simulink model "roll1818002"  (R2022b)
settings: Solver=ode1  StartTime=0.0  StopTime=500  FixedStep=0.01  RelTol=1e-3
values from neighbouring files (symbols this model uses):
  Kp = 16.374    [roll201818002.m]
  Td = 0.01    [roll201818002.m]
  Ti = 150    [roll201818002.m]
settings Model: Creator=Wasif  LastModifiedBy=Wasif
settings SolverCC: ZeroCrossAlgorithm=Adaptive
settings DataIOCC: ReturnWorkspaceOutputs=off
settings DebuggingCC: IgnoredZcDiagnostic=none

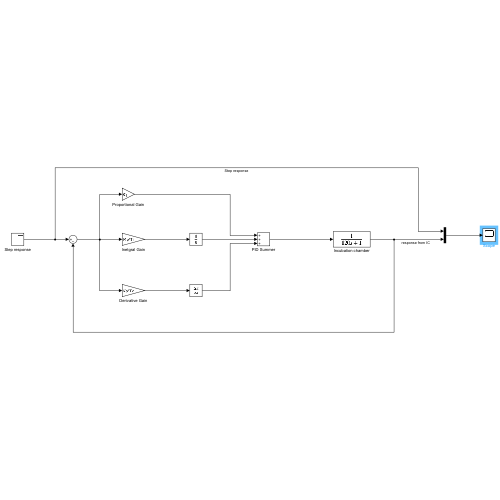
[thumbnail: Simulink's stored preview of the top-level diagram]
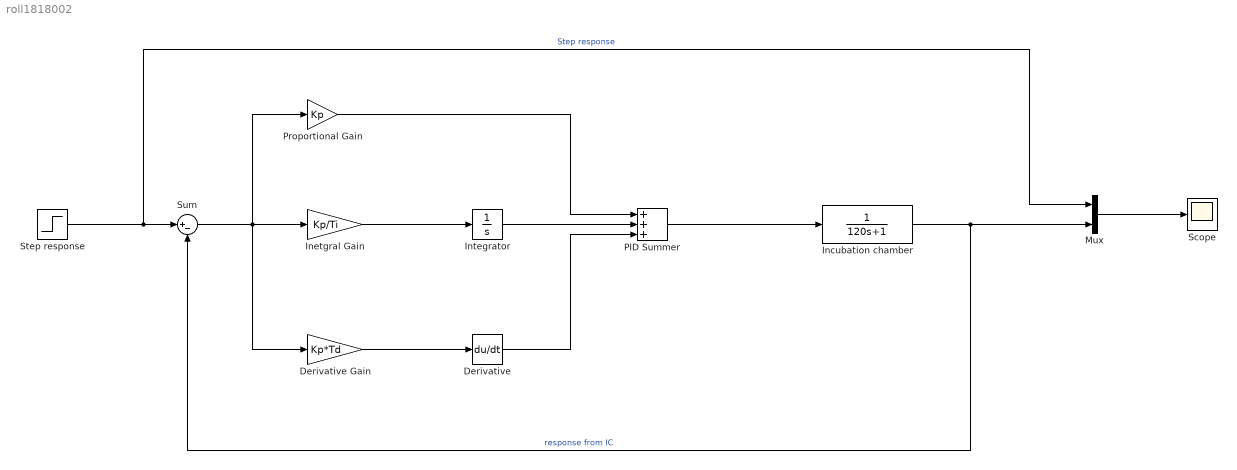
== system roll1818002 ==
  Derivative : Derivative
  Derivative Gain : Gain  Gain=Kp*Td
  Incubation chamber : TransferFcn  Denominator=[120 1]
  Inetgral Gain : Gain  Gain=Kp/Ti
  Integrator : Integrator
  Mux : Mux  Inputs=2
  PID Summer : Sum  Inputs=+++
  Proportional Gain : Gain  Gain=Kp
  Scope : Scope
  Step response : Step  SampleTime=0
  Sum : Sum  Inputs=|+-
  wires:
  Step response/1 -> Mux/1, Sum/1  "Step response"
  Sum/1 -> Derivative Gain/1, Inetgral Gain/1, Proportional Gain/1
  Derivative Gain/1 -> Derivative/1
  Inetgral Gain/1 -> Integrator/1
  Proportional Gain/1 -> PID Summer/1
  Integrator/1 -> PID Summer/2
  Derivative/1 -> PID Summer/3
  Incubation chamber/1 -> Mux/2, Sum/2  "response from IC"
  Mux/1 -> Scope/1
  PID Summer/1 -> Incubation chamber/1
